simulink model "TRU_debugg"  (R2013a)
settings: Solver=ode45  StartTime=0.0  StopTime=1000  RelTol=1e-3
libraries: simulink x1, powerlib_meascontrol x1, PowerFlowLib x1
settings Model: Creator=Bradford  LastModifiedBy=Bradford

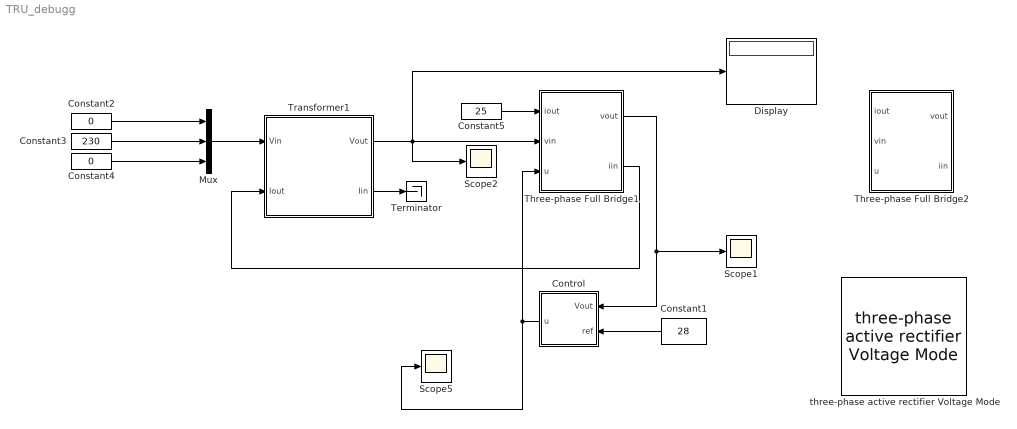
== system TRU_debugg ==
  Constant1 : Constant  Value=28
  Constant2 : Constant  Value=0
  Constant3 : Constant  Value=230
  Constant4 : Constant  Value=0
  Constant5 : Constant  Value=25
  Control : Subsystem
  Display : Display
  Mux : Mux  Inputs=3
  Scope1 : Scope
      settings: YMin=-32.49361  YMax=4.72151
  Scope2 : Scope
      settings: ShowLegends=on  YMin=-32.49361  YMax=4.72151  SaveName=ScopeData2
  Scope5 : Scope
      settings: YMin=-32.49361  YMax=4.72151
  Terminator : Terminator
  Three-phase Full Bridge1 : Subsystem  AncestorBlock=PowerFlowLib/Energy & Power Systems/Electrical/Rectifiers/Three-phase Full Bridge1  mask(Single-phase full bridge rectifier.){C=100e-6, Rc=1}
      mask prompts: C "Output capacitance (F):"; Rc "Circuit parasitic resistance (ohm):"
      mask help: Single-phase Full bridge rectifier. Lead resistance is added to make simulation possible.
  Three-phase Full Bridge2 : Subsystem  AncestorBlock=PowerFlowLib/Energy & Power Systems/Electrical/Rectifiers/Three-phase Full Bridge1  mask(Single-phase full bridge rectifier.){C=100e-6, Rc=1}
      mask prompts: C "Output capacitance (F):"; Rc "Circuit parasitic resistance (ohm):"
      mask help: Single-phase Full bridge rectifier. Lead resistance is added to make simulation possible.
  Transformer1 : Subsystem  AncestorBlock=PowerFlowLib/Energy & Power Systems/Electrical/Machines/Transformer  mask(Transformer){Rp=0.005, Rs=0.1, N1=400, N2=45}
      mask prompts: Rp "Primary Winding Resistance"; Rs "Secondary Winding Resistance"; N1 "Number of Turns in Primary"; N2 "Number of Turns in Secondary"
      mask help:
      | The user inputs and outputs are given below. Inputs to the model are:
      |
      | Block Inputs
      | #1: Primary voltage input [V]
      | #2: Secondary current input [A]
      |
      | Block Outputs
      | #1: Secondary voltage output [V]
      | #2: Primary current input [A]
      mask Help: eval('open(''Transformer Help.html'')');
      mask Display:
      | image(imread('Transformer.png'))
      | 
      | port_label('input',1,'{\bf V_i_n}','TexMode','on')
      | port_label('input',2,'{\bf I_o_u_t}','TexMode','on')
      | 
      | port_label('output',1,'{\bf V_o_u_t}','TexMode','on')
      | port_label('output',2,'{\bf I_i_n}','TexMode','on')
  three-phase active rectifier Voltage Mode : PowerFlowLib/Energy & Power Systems/Electrical/Rectifiers/three-phase  active rectifier Voltage Mode  L=1e-3  C=1e-4
  wires:
  Three-phase Full Bridge1/1(vout) -> Scope1/1, Control/1(Vout)
  Constant5/1 -> Three-phase Full Bridge1/1(iout)
  Three-phase Full Bridge1/2(iin) -> Transformer1/2(Iout)
  Transformer1/1(Vout) -> Scope2/1, Display/1, Three-phase Full Bridge1/2(vin)
  Transformer1/2(Iin) -> Terminator/1
  Constant1/1 -> Control/2(ref)
  Control/1(u) -> Three-phase Full Bridge1/3(u), Scope5/1
  Mux/1 -> Transformer1/1(Vin)
  Constant2/1 -> Mux/1
  Constant3/1 -> Mux/2
  Constant4/1 -> Mux/3

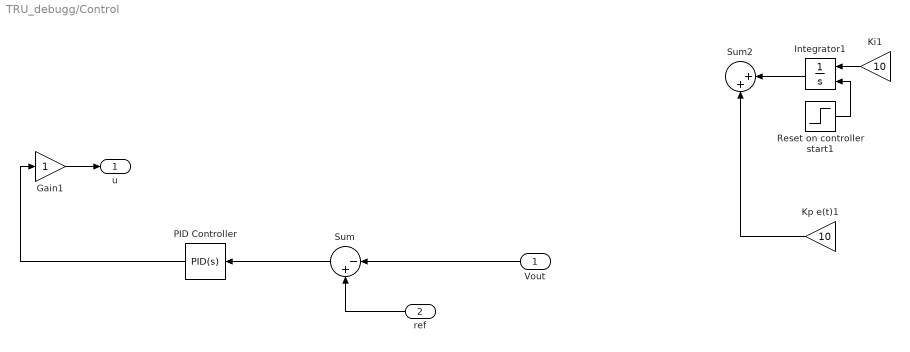
== system TRU_debugg/Control ==
  Vout : Inport
  ref : Inport  Port=2
  Gain1 : Gain
  Integrator1 : Integrator  ExternalReset=rising
  Ki1 : Gain  Gain=10
  Kp e(t)1 : Gain  Gain=10
  PID Controller : simulink/Continuous/PID Controller  Controller=PID  TimeDomain=Continuous-time  SampleTime=1  IntegratorMethod=Forward Euler  FilterMethod=Forward Euler  Form=Parallel  P=0  I=-20.0000452359282  D=0  N=100  InitialConditionSource=internal  InitialConditionForIntegrator=0  InitialConditionForFilter=0  ExternalReset=none  LimitOutput=off  UpperSaturationLimit=inf  LowerSaturationLimit=-inf  LinearizeAsGain=on  AntiWindupMode=none  Kb=1  TrackingMode=off  Kt=1  PParamMin=[]  PParamMax=[]  IParamMin=[]  IParamMax=[]  DParamMin=[]  DParamMax=[]  NParamMin=[]  NParamMax=[]  KbParamMin=[]  KbParamMax=[]  KtParamMin=[]  KtParamMax=[]  POutMin=[]  POutMax=[]  IOutMin=[]  IOutMax=[]  DOutMin=[]  DOutMax=[]  NOutMin=[]  NOutMax=[]  KbOutMin=[]  KbOutMax=[]  KtOutMin=[]  KtOutMax=[]  IntegratorOutMin=[]  IntegratorOutMax=[]  FilterOutMin=[]  FilterOutMax=[]  SumOutMin=[]  SumOutMax=[]  SumI1OutMin=[]  SumI1OutMax=[]  SumI2OutMin=[]  SumI2OutMax=[]  SumI3OutMin=[]  SumI3OutMax=[]  SumDOutMin=[]  SumDOutMax=[]  SaturationOutMin=[]  SaturationOutMax=[]  IntegratorContinuousStateAttributes=''  IntegratorStateMustResolveToSignalObject=off  IntegratorRTWStateStorageClass=Auto  FilterContinuousStateAttributes=''  FilterStateMustResolveToSignalObject=off  FilterRTWStateStorageClass=Auto
  Reset on controller start1 : Step  Time=75  SampleTime=0
  Sum : Sum  Inputs=|-+
  Sum2 : Sum  Inputs=|++
  u : Outport
  wires:
  PID Controller/1 -> Gain1/1
  Vout/1 -> Sum/1
  ref/1 -> Sum/2
  Gain1/1 -> u/1
  ? -> Ki1/1, Kp e(t)1/1
  Reset on controller start1/1 -> Integrator1/2
  Ki1/1 -> Integrator1/1
  Kp e(t)1/1 -> Sum2/2
  Integrator1/1 -> Sum2/1
  Sum/1 -> PID Controller/1

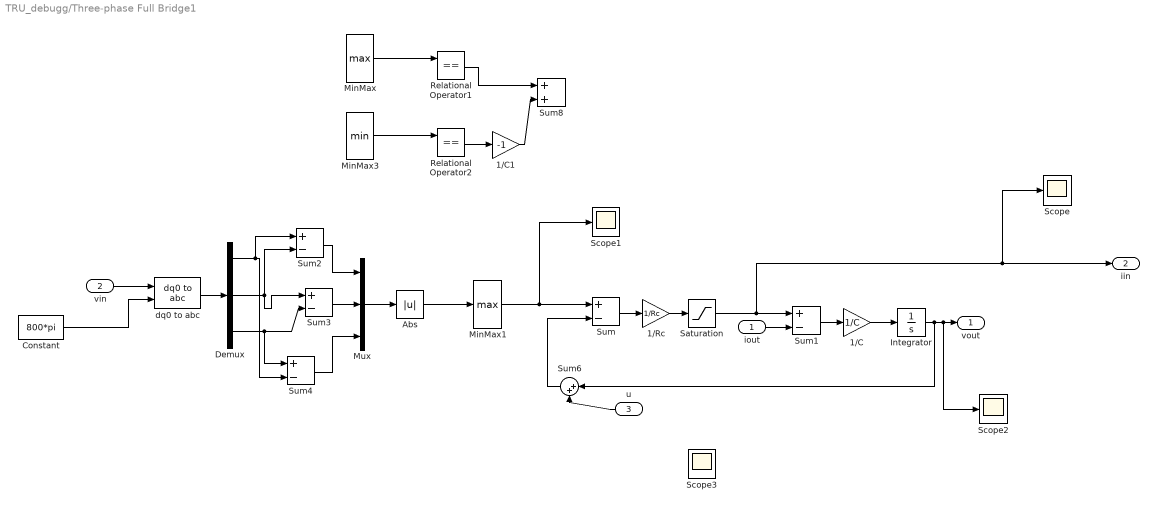
== system TRU_debugg/Three-phase Full Bridge1 ==
  iout : Inport
  vin : Inport  Port=2
  u : Inport  Port=3
  1/C : Gain  Gain=1/C  SaturateOnIntegerOverflow=on  OutDataTypeStr=Inherit: Same as input  ParamDataTypeStr=Inherit: Same as input
  1/C1 : Gain  Gain=-1  SaturateOnIntegerOverflow=on  OutDataTypeStr=Inherit: Same as input  ParamDataTypeStr=Inherit: Same as input
  1/Rc : Gain  Gain=1/Rc  SaturateOnIntegerOverflow=on  OutDataTypeStr=Inherit: Same as input  ParamDataTypeStr=Inherit: Same as input
  Abs : Abs  SaturateOnIntegerOverflow=on
  Constant : Constant  Value=800*pi
  Demux : Demux  Outputs=3
  Integrator : Integrator  InitialCondition=20
  MinMax : MinMax  Function=max
  MinMax1 : MinMax  Function=max
  MinMax3 : MinMax
  Mux : Mux  Inputs=3
  Relational Operator1 : RelationalOperator  Operator===  OutDataTypeStr=float('double')
  Relational Operator2 : RelationalOperator  Operator===  OutDataTypeStr=float('double')
  Saturation : Saturate  UpperLimit=inf  LowerLimit=0
  Scope{,1..3} (4 alike) : Scope
      Scope settings: YMin=-3.32249  YMax=29.90241  SaveName=ScopeData12
      Scope1 settings: YMin=-3.32249  YMax=29.90241  SaveName=ScopeData3
      Scope2 settings: YMin=-3.32249  YMax=29.90241  SaveName=ScopeData5
      Scope3 settings: YMin=-3.32249  YMax=29.90241  SaveName=ScopeData6
  Sum{,1..4} (5 alike) : Sum  Inputs=+-  SaturateOnIntegerOverflow=on  InputSameDT=on  OutDataTypeStr=Inherit: Same as first input
  Sum6 : Sum  Inputs=|++
  Sum8 : Sum  OutDataTypeStr=double  SaturateOnIntegerOverflow=on
  dq0 to abc : powerlib_meascontrol/Transformations/dq0 to abc  Alignment=90 degrees behind phase A axis
  vout : Outport
  iin : Outport  Port=2
  wires:
  1/C1/1 -> Sum8/2
  Relational Operator2/1 -> 1/C1/1
  Relational Operator1/1 -> Sum8/1
  MinMax3/1 -> Relational Operator2/1
  MinMax/1 -> Relational Operator1/1
  Sum4/1 -> Mux/3
  Sum3/1 -> Mux/2
  Sum2/1 -> Mux/1
  Demux/3 -> Sum4/1, Sum3/2
  Demux/2 -> Sum2/2, Sum3/1
  Demux/1 -> Sum4/2, Sum2/1
  Abs/1 -> MinMax1/1
  Mux/1 -> Abs/1
  Saturation/1 -> iin/1, Scope/1, Sum1/1
  Sum/1 -> 1/Rc/1
  iout/1 -> Sum1/2
  1/Rc/1 -> Saturation/1
  Integrator/1 -> Sum6/1, Scope2/1, vout/1
  Sum1/1 -> 1/C/1
  1/C/1 -> Integrator/1
  MinMax1/1 -> Scope1/1, Sum/1
  vin/1 -> dq0 to abc/1
  dq0 to abc/1 -> Demux/1
  Constant/1 -> dq0 to abc/2
  Sum6/1 -> Sum/2
  u/1 -> Sum6/2

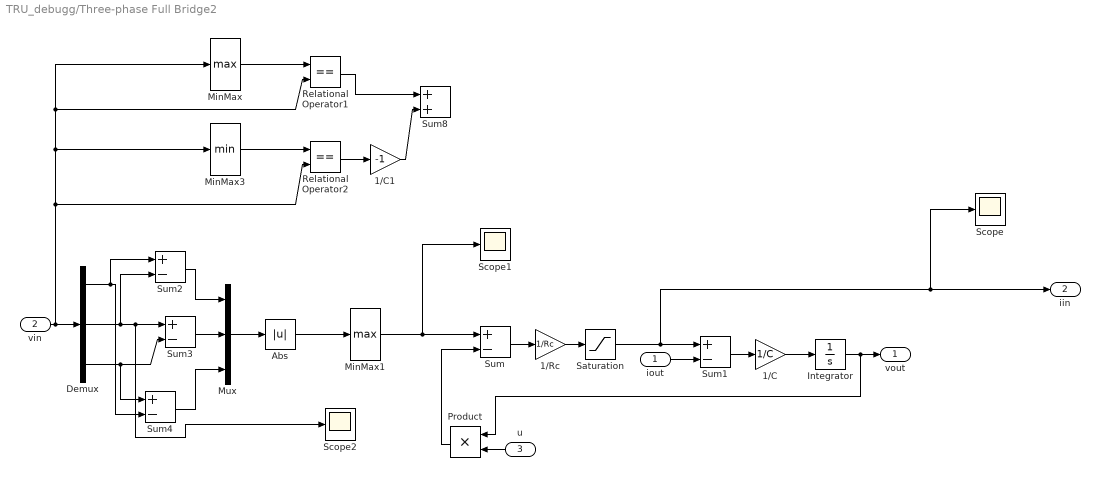
== system TRU_debugg/Three-phase Full Bridge2 ==
  iout : Inport
  vin : Inport  Port=2
  u : Inport  Port=3
  1/C : Gain  Gain=1/C  SaturateOnIntegerOverflow=on  OutDataTypeStr=Inherit: Same as input  ParamDataTypeStr=Inherit: Same as input
  1/C1 : Gain  Gain=-1  SaturateOnIntegerOverflow=on  OutDataTypeStr=Inherit: Same as input  ParamDataTypeStr=Inherit: Same as input
  1/Rc : Gain  Gain=1/Rc  SaturateOnIntegerOverflow=on  OutDataTypeStr=Inherit: Same as input  ParamDataTypeStr=Inherit: Same as input
  Abs : Abs  SaturateOnIntegerOverflow=on
  Demux : Demux  Outputs=3
  Integrator : Integrator  InitialCondition=20
  MinMax : MinMax  Function=max
  MinMax1 : MinMax  Function=max
  MinMax3 : MinMax
  Mux : Mux  Inputs=3
  Product : Product
  Relational Operator1 : RelationalOperator  Operator===  OutDataTypeStr=float('double')
  Relational Operator2 : RelationalOperator  Operator===  OutDataTypeStr=float('double')
  Saturation : Saturate  UpperLimit=inf  LowerLimit=0
  Scope : Scope
      settings: YMin=-3.32249  YMax=29.90241  SaveName=ScopeData12
  Scope1 : Scope
      settings: YMin=-3.32249  YMax=29.90241  SaveName=ScopeData3
  Scope2 : Scope
      settings: YMin=-3.32249  YMax=29.90241  SaveName=ScopeData4
  Sum{,1..4} (5 alike) : Sum  Inputs=+-  SaturateOnIntegerOverflow=on  InputSameDT=on  OutDataTypeStr=Inherit: Same as first input
  Sum8 : Sum  OutDataTypeStr=double  SaturateOnIntegerOverflow=on
  vout : Outport
  iin : Outport  Port=2
  wires:
  MinMax1/1 -> Sum/1, Scope1/1
  1/C/1 -> Integrator/1
  Sum1/1 -> 1/C/1
  Integrator/1 -> vout/1, Product/1
  1/Rc/1 -> Saturation/1
  iout/1 -> Sum1/2
  Sum/1 -> 1/Rc/1
  Saturation/1 -> Sum1/1, Scope/1, iin/1
  vin/1 -> MinMax/1, Relational Operator1/2, MinMax3/1, Relational Operator2/2, Demux/1
  Mux/1 -> Abs/1
  Abs/1 -> MinMax1/1
  Demux/1 -> Sum2/1, Sum4/2
  Demux/2 -> Sum3/1, Scope2/1, Sum2/2
  Demux/3 -> Sum3/2, Sum4/1
  Sum2/1 -> Mux/1
  Sum3/1 -> Mux/2
  Sum4/1 -> Mux/3
  MinMax/1 -> Relational Operator1/1
  MinMax3/1 -> Relational Operator2/1
  Relational Operator1/1 -> Sum8/1
  Relational Operator2/1 -> 1/C1/1
  1/C1/1 -> Sum8/2
  u/1 -> Product/2
  Product/1 -> Sum/2

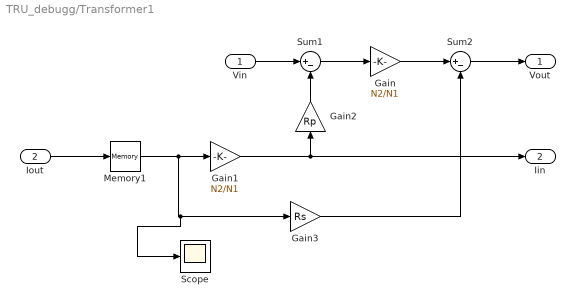
== system TRU_debugg/Transformer1 ==
  Vin : Inport
  Iout : Inport  Port=2
  Gain : Gain  Gain=N2/N1
  Gain1 : Gain  Gain=N2/N1
  Gain2 : Gain  Gain=Rp
  Gain3 : Gain  Gain=Rs
  Memory1 : Memory
  Scope : Scope
      settings: YMin=-1.03024  YMax=9.27213  SaveName=ScopeData11
  Sum1 : Sum  Inputs=|+-
  Sum2 : Sum  Inputs=|+-
  Vout : Outport
  Iin : Outport  Port=2
  wires:
  Memory1/1 -> Gain1/1, Gain3/1, Scope/1
  Iout/1 -> Memory1/1
  Vin/1 -> Sum1/1
  Gain2/1 -> Sum1/2
  Sum1/1 -> Gain/1
  Gain/1 -> Sum2/1
  Sum2/1 -> Vout/1
  Gain1/1 -> Gain2/1, Iin/1
  Gain3/1 -> Sum2/2
